simulink model "dllModel"  (R2022b)
settings: Solver=ode1  StartTime=0.0  StopTime=1145  FixedStep=0.001  RelTol=1e-3  EnableMultiTasking=on
values from neighbouring files (symbols this model uses):
  InputSignal = Simulink.Parameter    [dllModel_RAM_ROM.m]
settings Model: SimulationMode=accelerator  Creator=C3038028  LastModifiedBy=OMEN
settings SolverCC: AlgebraicLoopSolver=TrustRegion
settings DataIOCC: SaveOutput=off  SignalLogging=off  VisualizeSimOutput=off  SaveTime=off  ReturnWorkspaceOutputs=off
settings OptimizationCC: BlockReduction=off  ConditionallyExecuteInputs=off  DefaultParameterBehavior=Inlined  DefaultUnderspecifiedDataType=single  LifeSpan=Inf  EfficientTunableParamExpr=on
settings DebuggingCC: UnconnectedInputMsg=warning  UnconnectedOutputMsg=warning  UnconnectedLineMsg=warning  AllowSymbolicDim=off  SFUnexpectedBacktrackingDiag=warning  SFNoUnconditionalDefaultTransitionDiag=warning  SFExecutionAtInitializationDiag=none  SFMachineParentedDataDiag=warning  ArithmeticOperatorsInVariantConditions=warning
settings HardwareCC: TargetBitPerPointer=64  TargetBitPerSizeT=64  TargetBitPerPtrDiffT=64  TargetLongLongMode=on  TargetIntDivRoundTo=Zero  TargetEndianess=LittleEndian  TargetWordSize=64  TargetHWDeviceType=MATLAB Host  ProdEqTarget=off
settings ModelReferenceCC: EnableRefExpFcnMdlSchedulingChecks=on  PropagateSignalLabelsOutOfModel=off
settings SFSimCC: SimUseLocalCustomCode=off  MATLABDynamicMemAlloc=off  CustomCodeUndefinedFunction=UseInterfaceOnly
settings RTWCC: Description=Embedded Coder (host-based shared library target)  SystemTargetFile=ert_shrlib.tlc  TemplateMakefile=ert_default_tmf  RTWUseLocalCustomCode=off  BuildConfiguration=Faster Runs
settings CodeAppCC: IgnoreCustomStorageClasses=off  StateflowObjectComments=on
settings STFCustomTargetCC: GenerateSampleERTMain=on  ParMdlRefBuildCompliant=on  CompOptLevelCompliant=on  CombineOutputUpdateFcns=on  ERTCustomFileBanners=on  SupportNonInlinedSFcns=off  RemoveResetFunc=on  MATLABClassNameForMDSCustomization=Simulink.SoftwareTarget.ERTCustomization  ModelStepFunctionPrototypeControlCompliant=on  UseToolchainInfoCompliant=on  SystemTargetFile=ert_shrlib.tlc
settings ERTTargetCC: MultiwordLength=2048  GenerateSampleERTMain=on  ConcurrentExecutionCompliant=off  SupportContinuousTime=on  CPPClassGenCompliant=off  InlinedParameterPlacement=NonHierarchical  ERTCustomFileTemplate=example_file_process.tlc  ConvertIfToSwitch=off  SuppressUnreachableDefaultCases=off
settings ConfigComp: CovMetricSettings=dw  CovSaveCumulativeToWorkspaceVar=on  CovSaveSingleToWorkspaceVar=on  CovExternalEMLEnable=off

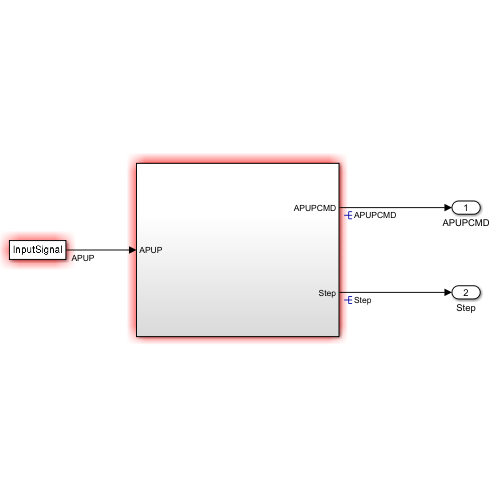
[thumbnail: Simulink's stored preview of the top-level diagram]
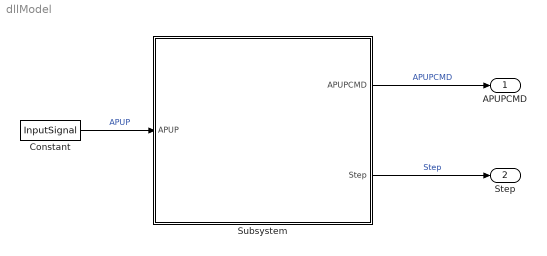
== system dllModel ==
  Constant : Constant  Value=InputSignal  OutDataTypeStr=double  SampleTime=0.001
  Subsystem : Subsystem
  APUPCMD : Outport  VectorParamsAs1DForOutWhenUnconnected=off
  Step : Outport  Port=2  VectorParamsAs1DForOutWhenUnconnected=off
  wires:
  Constant/1 -> Subsystem/1(APUP)  "APUP"
  Subsystem/1(APUPCMD) -> APUPCMD/1  "APUPCMD"
  Subsystem/2(Step) -> Step/1  "Step"

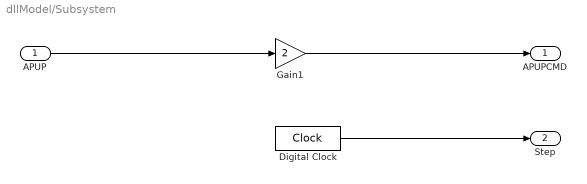
== system dllModel/Subsystem ==
  APUP : Inport
  Digital Clock : DigitalClock  SampleTime=0.001
  Gain1 : Gain  Gain=2
  APUPCMD : Outport  VectorParamsAs1DForOutWhenUnconnected=off
  Step : Outport  Port=2  VectorParamsAs1DForOutWhenUnconnected=off
  wires:
  Digital Clock/1 -> Step/1
  Gain1/1 -> APUPCMD/1
  APUP/1 -> Gain1/1
